simulink model "part3"  (R2015a)
settings: Solver=ode45  StartTime=0.0  StopTime=2  RelTol=1e-3
values from neighbouring files (symbols this model uses):
  kd3 = kp3*Td    [part3code.m]
  ki3 = kp3/Ti    [part3code.m]
  kp3 = 0.56878    [part3code.m]
settings Model: Creator=Γιώργος  LastModifiedBy=Γιώργος

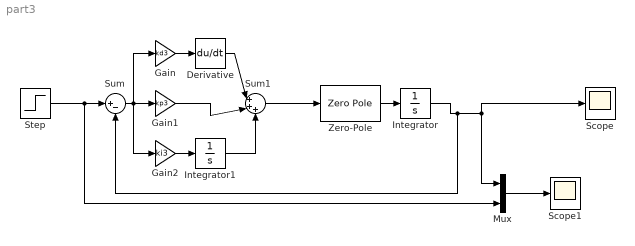
== system part3 ==
  Derivative : Derivative
  Gain : Gain  Gain=kd3
  Gain1 : Gain  Gain=kp3
  Gain2 : Gain  Gain=ki3
  Integrator : Integrator
  Integrator1 : Integrator
  Mux : Mux  Inputs=2
  Scope : Scope
  Scope1 : Scope
  Step : Step  SampleTime=0
  Sum : Sum  Inputs=|+-
  Sum1 : Sum  Inputs=|+++
  Zero-Pole : ZeroPole  Zeros=[0]  Poles="[0  -400.26 -3008]"  Gain=[2.717*10^9]
  wires:
  Sum/1 -> Gain/1, Gain2/1, Gain1/1
  Step/1 -> Mux/2, Sum/1
  Mux/1 -> Scope1/1
  Zero-Pole/1 -> Integrator/1
  Integrator/1 -> Sum/2, Mux/1, Scope/1
  Gain2/1 -> Integrator1/1
  Gain/1 -> Derivative/1
  Derivative/1 -> Sum1/1
  Gain1/1 -> Sum1/2
  Integrator1/1 -> Sum1/3
  Sum1/1 -> Zero-Pole/1
